simulink subsystem "Triangle_Reference"  (R2022b)
settings: Solver=VariableStepAuto  StartTime=0.0  StopTime=10.0  RelTol=1e-3
model mask{Freq=1, Gain=1, Value=0}
  mask prompts: Freq "Frequency (Hz):"; Gain "Amplitude:"; Value "Bias:"
libraries: spsTriangleGeneratorLib x1
settings Model: Creator=gotta  LastModifiedBy=gotta

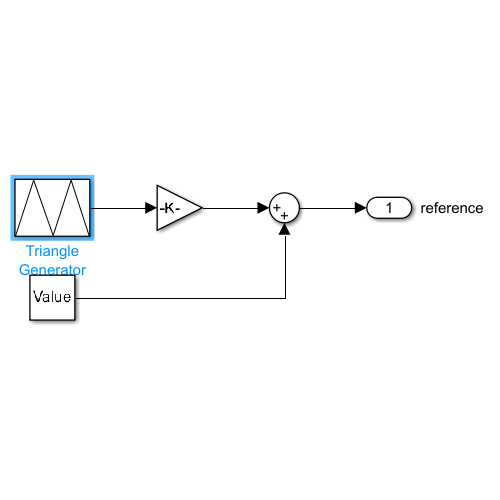
[thumbnail: Simulink's stored preview of the top-level diagram]
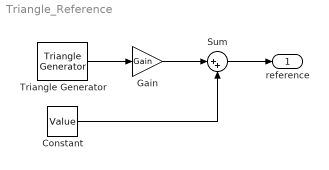
== system Triangle_Reference ==
  Constant : Constant  Value=Value
  Gain : Gain  Gain=Gain
  Sum : Sum  Inputs=|++
  Triangle Generator : spsTriangleGeneratorLib/Triangle Generator  Freq=Freq  Phase=90  Ts=0
  reference : Outport
  wires:
  Triangle Generator/1 -> Gain/1
  Gain/1 -> Sum/1
  Constant/1 -> Sum/2
  Sum/1 -> reference/1
